simulink model "simulink_sfbk_R2018a"  (R2018a)
settings: Solver=ode4  StartTime=0.0  StopTime=4  FixedStep=0.01  RelTol=1e-3  EnableMultiTasking=on
values from neighbouring files (symbols this model uses):
  A = [  0  1 ... (first row only)    [optimal_care.m]    (also in optimal_hamilton.m; optimal_hamilton2.m; optimal_lqr.m; optimal_servo.m = [ 0  1  0  0)
  B = [ 0 ... (first row only)    [optimal_care.m]    (also in optimal_hamilton.m; optimal_hamilton2.m; optimal_lqr.m; optimal_servo.m)
  K = - inv(R)*B'*P    [optimal_care.m]    (also in optimal_lqr.m = - lqr(A,B,Q,R); optimal_servo.m = - inv(Re)*B'*P11; symb_riccati.m = double(K))
  x0 = [ 1  0 ]'    [run_simulink_lqr.m]    (also in run_simulink_optimal_servo.m = [ 0  0  0.25  0 ]')
settings Model: Creator=kawata  LastModifiedBy=kawata
settings DataIOCC: LimitDataPoints=on  SaveFormat=Array  SignalLoggingSaveFormat=ModelDataLogs
settings OptimizationCC: ExpressionDepthLimit=2147483647  LifeSpan=inf
settings DebuggingCC: UnderspecifiedInitializationDetection=Classic  MergeDetectMultiDrivingBlocksExec=none  SolverPrmCheckMsg=warning  FcnCallInpInsideContextMsg=warning  StateNameClashWarn=warning  SFUnexpectedBacktrackingDiag=warning  SFNoUnconditionalDefaultTransitionDiag=warning  SFExecutionAtInitializationDiag=none
settings HardwareCC: ProdBitPerPointer=32  ProdBitPerSizeT=32  ProdBitPerPtrDiffT=32  ProdLargestAtomicFloat=None  ProdIntDivRoundTo=Undefined  ProdEndianess=Unspecified  ProdWordSize=32  ProdHWDeviceType=32-bit Generic
settings ModelReferenceCC: PropagateSignalLabelsOutOfModel=off
settings CodeAppCC: StateflowObjectComments=on
settings GRTTargetCC: TargetLangStandard=C89/C90 (ANSI)  GeneratePreprocessorConditionals=Disable all  CombineOutputUpdateFcns=off  GRTInterface=on
settings ConfigComp: CovMetricSettings=dw  CovHtmlReporting=on  CovSaveCumulativeToWorkspaceVar=on  CovSaveSingleToWorkspaceVar=on  CovExternalEMLEnable=off

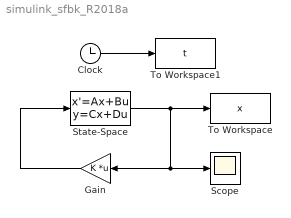
== system simulink_sfbk_R2018a ==
  Clock : Clock
  Gain : Gain  Gain=K  Multiplication=Matrix(K*u)
  Scope : Scope
  State-Space : StateSpace  A=A  B=B  C=eye(2)  D=zeros(2,1)  InitialCondition=x0
  To Workspace : ToWorkspace  VariableName=x  SampleTime=-1
  To Workspace1 : ToWorkspace  VariableName=t  SampleTime=-1
  wires:
  State-Space/1 -> Gain/1, Scope/1, To Workspace/1
  Clock/1 -> To Workspace1/1
  Gain/1 -> State-Space/1
